simulink model "Inverters_Data"  (R2023b)
settings: Solver=FixedStepAuto  StartTime=0.0  StopTime=10.0  RelTol=1e-3
libraries: simulink x3
settings Model: Creator=cspt  LastModifiedBy=joser
settings SolverCC: AlgebraicLoopSolver=TrustRegion
settings DataIOCC: SaveOutput=off  ReturnWorkspaceOutputs=off
settings OptimizationCC: DefaultParameterBehavior=Inlined
settings DebuggingCC: UnconnectedInputMsg=warning  UnconnectedOutputMsg=warning  UnconnectedLineMsg=warning  ArithmeticOperatorsInVariantConditions=warning
settings ModelReferenceCC: EnableRefExpFcnMdlSchedulingChecks=on
settings SFSimCC: SimUseLocalCustomCode=off  CustomCodeUndefinedFunction=UseInterfaceOnly
settings RTWCC: Description=INTECRIO Real-Time Target  SystemTargetFile=irt.tlc  TemplateMakefile=irt_default_tmf  RTWUseLocalCustomCode=off
settings STFCustomTargetCC: UtilityFuncGeneration=Shared location  MatFileLogging=on  GRTInterface=on  SystemTargetFile=irt.tlc
settings GRTTargetCC: UtilityFuncGeneration=Shared location  ParMdlRefBuildCompliant=off  CompOptLevelCompliant=off  ConcurrentExecutionCompliant=off  CombineOutputUpdateFcns=off  CPPClassGenCompliant=off  GRTInterface=on  UseToolchainInfoCompliant=off  GenerateASAP2=on

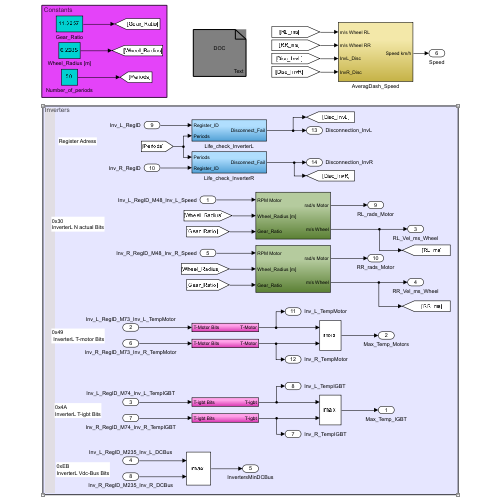
[thumbnail: Simulink's stored preview of the top-level diagram]
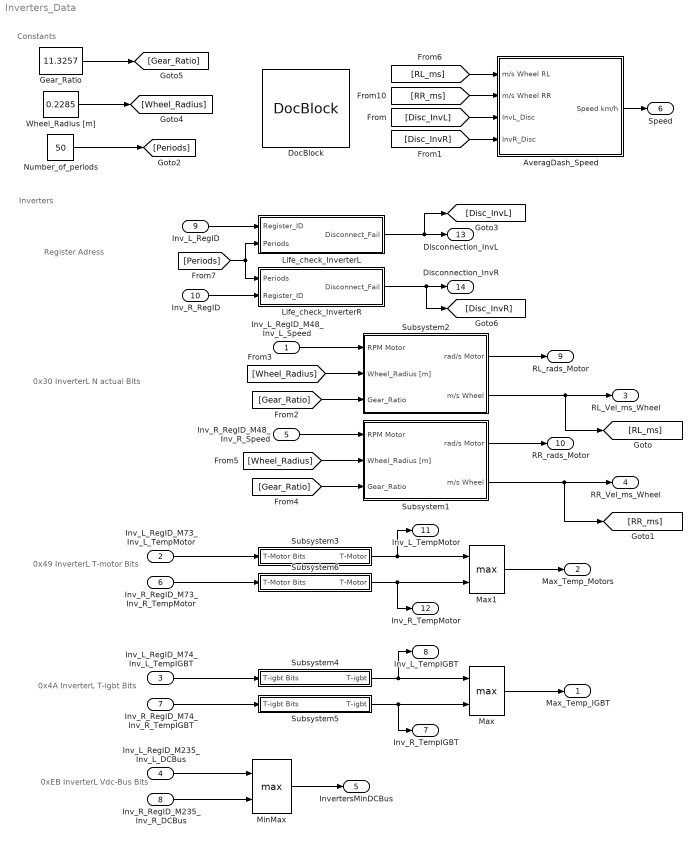
== system Inverters_Data ==
  note: Constants
  note: 0x49
      |  InverterL T-motor Bits
  note: 0x4A
      | InverterL T-igbt Bits
  note: 0xEB
      | InverterL Vdc-Bus Bits
  note: 0x30
      | InverterL N actual Bits
  note: Inverters
  note: Register Adress
  Inv_L_RegID_M48_Inv_L_Speed : Inport
  Inv_L_RegID_M73_Inv_L_TempMotor : Inport  Port=2
  Inv_L_RegID_M74_Inv_L_TempIGBT : Inport  Port=3
  Inv_L_RegID_M235_Inv_L_DCBus : Inport  Port=4
  Inv_R_RegID_M48_Inv_R_Speed : Inport  Port=5
  Inv_R_RegID_M73_Inv_R_TempMotor : Inport  Port=6
  Inv_R_RegID_M74_Inv_R_TempIGBT : Inport  Port=7
  Inv_R_RegID_M235_Inv_R_DCBus : Inport  Port=8
  Inv_L_RegID : Inport  Port=9
  Inv_R_RegID : Inport  Port=10
  AveragDash_Speed : Subsystem
  DocBlock : simulink/Model-Wide Utilities/DocBlock  DocumentType=Text
      content=|
      | Our Bamocar Inverters communicate with the environment in bits.
      | A maximum number of bits (32767) is selected to correspond to a maximum
      | number of current, RPM, etc., which would be equivalent to 100%, but it
      | can send or receive a greater number of bits.
      |
      | The 3 currents (Iq, Iactual, Icmd) conversion are done on the Database:
      | 400 / 1070 = 0.3738317757...
      |
      | The "Inv_X_DCBus" conversion is done on the Database: 0.03125
      | The function of Bits - VoltageDCBus is linear, so we need the slope:
      | f(Bits) = Voltage    f(22000 Bits) = 700 V     f(14000 Bits) = 450 V
      | (700 - 450) / (22000 - 14000) = 0.03125
      |
      | The "Inv_X_Speed" conversion is done on the Database:
      | 'N-100%' (RPMmax) / 32767 (Bits_max) = 0.18311057
      | RPMmax is the speed limit selected on the N-Drive Software (talk with Powertrain)
      |
      | The Motor Temp is done in the Database: TempM * 0.03282 - 114.92892
      |
      | The IGBT & Motor Temps are complex, so the conversions are done on the
      | Simulink. The Powertrain Department provided us with a Bits - Temp lookup
      | table. The Bits are on CAN1 (send by the Inverters) and the ºC are send
      | through CAN2.
      |
      | All values with understandable units are at CAN1, Message:
      | AP_Inverter_X_Tx (0xB5 & 0xB6),
      | but the IGBT & Motor Temps (ºC) are at CAN2:
      | MEAS_ETAS_Inverter_X_Data (0xD2 & 0xD3).
  Gear_Ratio : Constant  Value=11.3257
  Life_check_InverterL : Subsystem
  Life_check_InverterR : Subsystem
  Max : MinMax  Function=max  Inputs=2
  Max1 : MinMax  Function=max  Inputs=2
  MinMax : MinMax  Function=max  Inputs=2
  Number_of_periods : Constant  Value=50
  Subsystem1 : Subsystem
  Subsystem2 : Subsystem
  Subsystem3 : Subsystem
  Subsystem4 : Subsystem
  Subsystem5 : Subsystem
  Subsystem6 : Subsystem
  Wheel_Radius [m] : Constant  Value=0.2285
  Max_Temp_IGBT : Outport  VectorParamsAs1DForOutWhenUnconnected=off
  Max_Temp_Motors : Outport  Port=2  VectorParamsAs1DForOutWhenUnconnected=off
  RL_Vel_ms_Wheel : Outport  Port=3  VectorParamsAs1DForOutWhenUnconnected=off
  RR_Vel_ms_Wheel : Outport  Port=4  VectorParamsAs1DForOutWhenUnconnected=off
  InvertersMinDCBus : Outport  Port=5  VectorParamsAs1DForOutWhenUnconnected=off
  Speed : Outport  Port=6  VectorParamsAs1DForOutWhenUnconnected=off
  Inv_R_TempIGBT : Outport  Port=7  VectorParamsAs1DForOutWhenUnconnected=off
  Inv_L_TempIGBT : Outport  Port=8  VectorParamsAs1DForOutWhenUnconnected=off
  RL_rads_Motor : Outport  Port=9  VectorParamsAs1DForOutWhenUnconnected=off
  RR_rads_Motor : Outport  Port=10  VectorParamsAs1DForOutWhenUnconnected=off
  Inv_L_TempMotor : Outport  Port=11
  Inv_R_TempMotor : Outport  Port=12
  Disconnection_InvL : Outport  Port=13  VectorParamsAs1DForOutWhenUnconnected=off
  Disconnection_InvR : Outport  Port=14  VectorParamsAs1DForOutWhenUnconnected=off
  wires:
  Max1/1 -> Max_Temp_Motors/1
  [RR_ms] -> AveragDash_Speed/2(m/s Wheel RR)
  Subsystem2/2(m/s Wheel) -> [RL_ms], RL_Vel_ms_Wheel/1
  Subsystem4/1(T-igbt) -> Inv_L_TempIGBT/1, Max/1
  Subsystem1/2(m/s Wheel) -> RR_Vel_ms_Wheel/1, [RR_ms]
  Inv_L_RegID_M74_Inv_L_TempIGBT/1 -> Subsystem4/1(T-igbt Bits)
  [RL_ms] -> AveragDash_Speed/1(m/s Wheel RL)
  AveragDash_Speed/1(Speed km/h) -> Speed/1
  MinMax/1 -> InvertersMinDCBus/1
  Inv_R_RegID_M74_Inv_R_TempIGBT/1 -> Subsystem5/1(T-igbt Bits)
  Max/1 -> Max_Temp_IGBT/1
  Subsystem5/1(T-igbt) -> Inv_R_TempIGBT/1, Max/2
  Inv_L_RegID_M235_Inv_L_DCBus/1 -> MinMax/1
  Inv_R_RegID_M235_Inv_R_DCBus/1 -> MinMax/2
  Subsystem1/1(rad/s Motor) -> RR_rads_Motor/1
  Subsystem2/1(rad/s Motor) -> RL_rads_Motor/1
  Wheel_Radius [m]/1 -> [Wheel_Radius]
  Gear_Ratio/1 -> [Gear_Ratio]
  Inv_R_RegID_M48_Inv_R_Speed/1 -> Subsystem1/1(RPM Motor)
  [Gear_Ratio] -> Subsystem2/3(Gear_Ratio)
  [Wheel_Radius] -> Subsystem2/2(Wheel_Radius [m])
  Inv_L_RegID_M48_Inv_L_Speed/1 -> Subsystem2/1(RPM Motor)
  [Gear_Ratio] -> Subsystem1/3(Gear_Ratio)
  [Wheel_Radius] -> Subsystem1/2(Wheel_Radius [m])
  Life_check_InverterR/1(Disconnect_Fail) -> Disconnection_InvR/1, [Disc_InvR]
  Life_check_InverterL/1(Disconnect_Fail) -> Disconnection_InvL/1, [Disc_InvL]
  Inv_L_RegID/1 -> Life_check_InverterL/1(Register_ID)
  Inv_R_RegID/1 -> Life_check_InverterR/2(Register_ID)
  [Periods] -> Life_check_InverterR/1(Periods), Life_check_InverterL/2(Periods)
  Number_of_periods/1 -> [Periods]
  Inv_L_RegID_M73_Inv_L_TempMotor/1 -> Subsystem3/1(T-Motor Bits)
  Subsystem3/1(T-Motor) -> Max1/1, Inv_L_TempMotor/1
  Subsystem6/1(T-Motor) -> Inv_R_TempMotor/1, Max1/2
  Inv_R_RegID_M73_Inv_R_TempMotor/1 -> Subsystem6/1(T-Motor Bits)
  [Disc_InvR] -> AveragDash_Speed/4(InvR_Disc)
  [Disc_InvL] -> AveragDash_Speed/3(InvL_Disc)

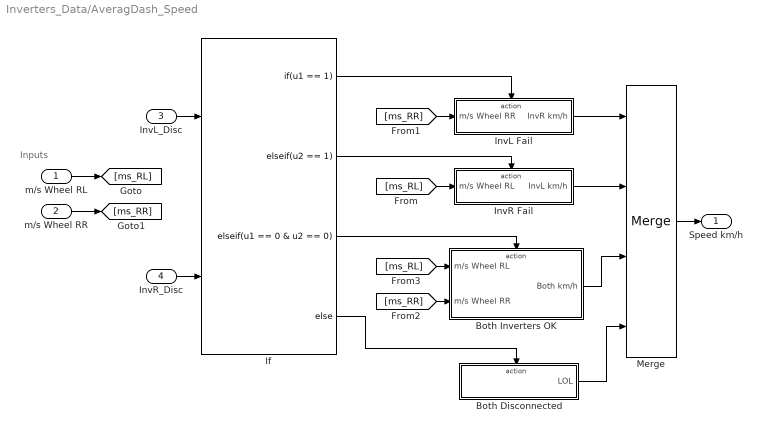
== system Inverters_Data/AveragDash_Speed ==
  note: Inputs
  m/s Wheel RL : Inport
  m/s Wheel RR : Inport  Port=2
  InvL_Disc : Inport  Port=3
  InvR_Disc : Inport  Port=4
  Both Disconnected : Subsystem  TreatAsAtomicUnit=on
  Both Inverters OK : Subsystem  TreatAsAtomicUnit=on
  If : If  NumInputs=2  IfExpression=u1 == 1  ElseIfExpressions=u2 == 1, u1 == 0 & u2 == 0
  InvL Fail : Subsystem  TreatAsAtomicUnit=on
  InvR Fail : Subsystem  TreatAsAtomicUnit=on
  Merge : Merge  Inputs=4
  Speed km/h : Outport  VectorParamsAs1DForOutWhenUnconnected=off
  wires:
  m/s Wheel RL/1 -> [ms_RL]
  m/s Wheel RR/1 -> [ms_RR]
  InvL_Disc/1 -> If/1
  InvR_Disc/1 -> If/2
  Merge/1 -> Speed km/h/1
  If/1 -> InvL Fail/Action
  If/2 -> InvR Fail/Action
  InvL Fail/1(InvR km/h) -> Merge/1
  InvR Fail/1(InvL km/h) -> Merge/2
  If/3 -> Both Inverters OK/Action
  Both Inverters OK/1(Both km/h) -> Merge/3
  [ms_RL] -> InvR Fail/1(m/s Wheel RL)
  [ms_RR] -> InvL Fail/1(m/s Wheel RR)
  [ms_RR] -> Both Inverters OK/2(m/s Wheel RR)
  [ms_RL] -> Both Inverters OK/1(m/s Wheel RL)
  If/4 -> Both Disconnected/Action
  Both Disconnected/1(LOL) -> Merge/4

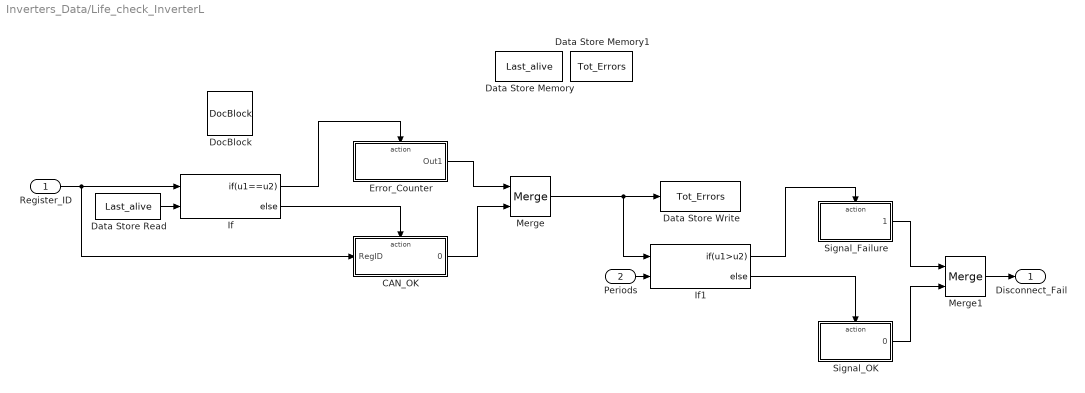
== system Inverters_Data/Life_check_InverterL ==
  Register_ID : Inport
  Periods : Inport  Port=2
  CAN_OK : Subsystem  TreatAsAtomicUnit=on
  Data Store Memory : DataStoreMemory  DataStoreName=Last_alive  ReadBeforeWriteMsg=warning  WriteAfterWriteMsg=warning  WriteAfterReadMsg=warning  ShowAdditionalParam=off
  Data Store Memory1 : DataStoreMemory  DataStoreName=Tot_Errors  ReadBeforeWriteMsg=warning  WriteAfterWriteMsg=warning  WriteAfterReadMsg=warning  ShowAdditionalParam=off
  Data Store Read : DataStoreRead  DataStoreName=Last_alive  IndexOptions=Index vector (dialog)  Indices=1  OutputSizes=1
  Data Store Write : DataStoreWrite  DataStoreName=Tot_Errors  IndexOptions=Index vector (dialog)  Indices=1  OutputSizes=1
  DocBlock : simulink/Model-Wide Utilities/DocBlock  DocumentType=Text
      content=|
      | The 'Inverters_Data' Simulink module is computed every 3ms by the ETAS.
      |
      | An Inverter is considered disconnected if the same value is obtained
      | from it for more than X seconds:
      | 0,003sec (Simulink computed) * P periods ('Periods' constant) = X seconds
      |
      | The Register Adress (RegID) has to modify its value every 3ms, because it
      | sends diferents signals every 3ms (multiplexed).
      |
      | This type of disconnection checks if there has been an error for more than
      | X seconds: STARTS counting since that first 'error' output. The important
      | thing about the Inverters' disconnections is the time it has been
      | disconnected, that's why we do it after checking the error.
      |
      | I've done some tests, and when I disconnect and then reconnect the
      | inverter, the RegID changes to a different period than before (3ms). I
      | don't understand why this happens.
      |
      | If we compute this subsystem at 'Disconnections', the ETAS would check the
      | alive every 25ms (when the RegID could be same as before), instead of every
      | 3ms (the RegID changes every 3ms).
      |
      | There's a an error -> Start counting errors -> Errors persist through X
      | periods -> Sensor disconnection
  Error_Counter : Subsystem  TreatAsAtomicUnit=on
  If : If  NumInputs=2  IfExpression=u1==u2
  If1 : If  NumInputs=2  IfExpression=u1>u2
  Merge : Merge
  Merge1 : Merge
  Signal_Failure : Subsystem  TreatAsAtomicUnit=on
  Signal_OK : Subsystem  TreatAsAtomicUnit=on
  Disconnect_Fail : Outport  VectorParamsAs1DForOutWhenUnconnected=off
  wires:
  Data Store Read/1 -> If/2
  If/2 -> CAN_OK/Action
  CAN_OK/1(0) -> Merge/2
  Register_ID/1 -> If/1, CAN_OK/1(RegID)
  If/1 -> Error_Counter/Action
  Error_Counter/1(Out1) -> Merge/1
  Merge/1 -> Data Store Write/1, If1/1
  If1/2 -> Signal_OK/Action
  Periods/1 -> If1/2
  Signal_Failure/1(1) -> Merge1/1
  If1/1 -> Signal_Failure/Action
  Signal_OK/1(0) -> Merge1/2
  Merge1/1 -> Disconnect_Fail/1

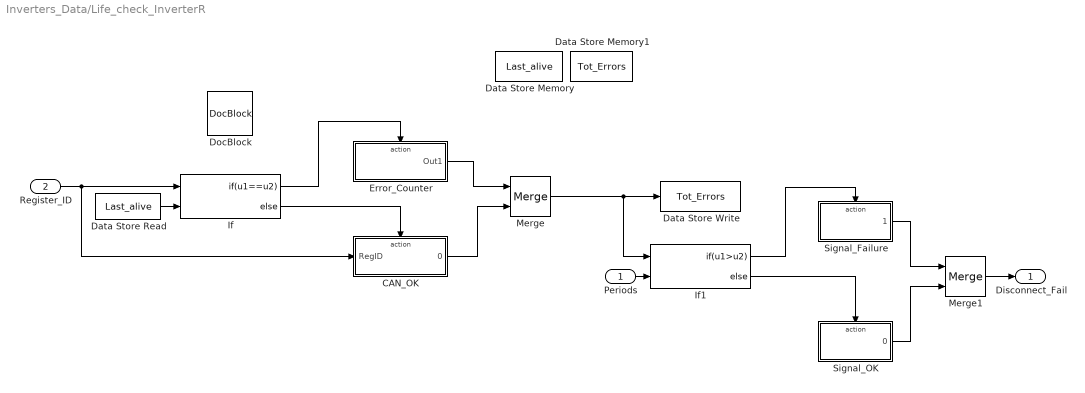
== system Inverters_Data/Life_check_InverterR ==
  Periods : Inport
  Register_ID : Inport  Port=2
  CAN_OK : Subsystem  TreatAsAtomicUnit=on
  Data Store Memory : DataStoreMemory  DataStoreName=Last_alive  ReadBeforeWriteMsg=warning  WriteAfterWriteMsg=warning  WriteAfterReadMsg=warning  ShowAdditionalParam=off
  Data Store Memory1 : DataStoreMemory  DataStoreName=Tot_Errors  ReadBeforeWriteMsg=warning  WriteAfterWriteMsg=warning  WriteAfterReadMsg=warning  ShowAdditionalParam=off
  Data Store Read : DataStoreRead  DataStoreName=Last_alive  IndexOptions=Index vector (dialog)  Indices=1  OutputSizes=1
  Data Store Write : DataStoreWrite  DataStoreName=Tot_Errors  IndexOptions=Index vector (dialog)  Indices=1  OutputSizes=1
  DocBlock : simulink/Model-Wide Utilities/DocBlock  DocumentType=Text
      content=|
      | The 'Inverters_Data' Simulink module is computed every 3ms by the ETAS.
      |
      | An Inverter is considered disconnected if the same value is obtained
      | from it for more than X seconds:
      | 0,003sec (Simulink computed) * P periods ('Periods' constant) = X seconds
      |
      | The Register Adress (RegID) has to modify its value every 3ms, because it
      | sends diferents signals every 3ms (multiplexed).
      |
      | This type of disconnection checks if there has been an error for more than
      | X seconds: STARTS counting since that first 'error' output. The important
      | thing about the Inverters' disconnections is the time it has been
      | disconnected, that's why we do it after checking the error.
      |
      | I've done some tests, and when I disconnect and then reconnect the
      | inverter, the RegID changes to a different period than before (3ms). I
      | don't understand why this happens.
      |
      | If we compute this subsystem at 'Disconnections', the ETAS would check the
      | alive every 25ms (when the RegID could be same as before), instead of every
      | 3ms (the RegID changes every 3ms).
      |
      | There's a an error -> Start counting errors -> Errors persist through X
      | periods -> Sensor disconnection
  Error_Counter : Subsystem  TreatAsAtomicUnit=on
  If : If  NumInputs=2  IfExpression=u1==u2
  If1 : If  NumInputs=2  IfExpression=u1>u2
  Merge : Merge
  Merge1 : Merge
  Signal_Failure : Subsystem  TreatAsAtomicUnit=on
  Signal_OK : Subsystem  TreatAsAtomicUnit=on
  Disconnect_Fail : Outport  VectorParamsAs1DForOutWhenUnconnected=off
  wires:
  Data Store Read/1 -> If/2
  If/2 -> CAN_OK/Action
  CAN_OK/1(0) -> Merge/2
  Register_ID/1 -> If/1, CAN_OK/1(RegID)
  If/1 -> Error_Counter/Action
  Error_Counter/1(Out1) -> Merge/1
  Merge/1 -> Data Store Write/1, If1/1
  If1/2 -> Signal_OK/Action
  Periods/1 -> If1/2
  Signal_Failure/1(1) -> Merge1/1
  If1/1 -> Signal_Failure/Action
  Signal_OK/1(0) -> Merge1/2
  Merge1/1 -> Disconnect_Fail/1

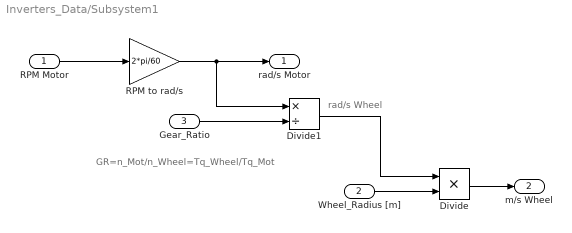
== system Inverters_Data/Subsystem1 ==
  note: rad/s Wheel
  note: GR=n_Mot/n_Wheel=Tq_Wheel/Tq_Mot
  RPM Motor : Inport
  Wheel_Radius [m] : Inport  Port=2
  Gear_Ratio : Inport  Port=3
  Divide : Product  Inputs=**
  Divide1 : Product  Inputs=*/
  RPM to rad/s : Gain  Gain=2*pi/60
  rad/s Motor : Outport  VectorParamsAs1DForOutWhenUnconnected=off
  m/s Wheel : Outport  Port=2
  wires:
  RPM to rad/s/1 -> Divide1/1, rad/s Motor/1
  Divide1/1 -> Divide/1
  Wheel_Radius [m]/1 -> Divide/2
  Divide/1 -> m/s Wheel/1
  Gear_Ratio/1 -> Divide1/2
  RPM Motor/1 -> RPM to rad/s/1

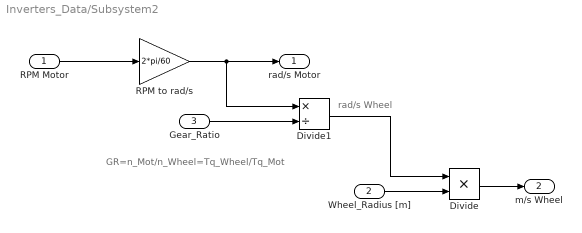
== system Inverters_Data/Subsystem2 ==
  note: rad/s Wheel
  note: GR=n_Mot/n_Wheel=Tq_Wheel/Tq_Mot
  RPM Motor : Inport
  Wheel_Radius [m] : Inport  Port=2
  Gear_Ratio : Inport  Port=3
  Divide : Product  Inputs=**
  Divide1 : Product  Inputs=*/
  RPM to rad/s : Gain  Gain=2*pi/60
  rad/s Motor : Outport  VectorParamsAs1DForOutWhenUnconnected=off
  m/s Wheel : Outport  Port=2
  wires:
  RPM to rad/s/1 -> Divide1/1, rad/s Motor/1
  Divide1/1 -> Divide/1
  Wheel_Radius [m]/1 -> Divide/2
  Divide/1 -> m/s Wheel/1
  Gear_Ratio/1 -> Divide1/2
  RPM Motor/1 -> RPM to rad/s/1

== system Inverters_Data/Subsystem3 ==
  T-Motor Bits : Inport
  1-D Lookup Table : Lookup_n-D  NumberOfTableDimensions=1  BreakpointsForDimension1=[3788.961224,3945.578464,4023.494666,4178.542234,4249.749706,4403.26785,4555.739546,4631.582976,4701.360096,4851.779144,5001.151744,5143.792394,5291.112346,5437.38585,5504.543754,5649.287834,5721.267456,5792.985466,5930.169416,6001.122714,6071.8144,6142.244474,6207.02465,6276.951624,6346.616986,6416.020736,6548.754186,6617.393224,6712,6816.5304,6868.5634,7075.1474,7126.4064,7228.46,7279.2546,7480.885,7530.9056,7580.7714,7680.0386,7729.44,7778.6866,7827.7784,7925.4976,7974.125,8022.5976,8119.0784,8262.6386,8357.5714,8404.8056,8592.1944,8638.6546,8822.9474,8914.165,9004.7634]  Table=[1.31,7.1,9.99,15.2,18.1,23.9,29.1,32,34.9,40.1,45.9,50.5,55.7,60.4,62.7,66.7,69,71.4,75.4,77.7,80,81.8,83.5,85.2,87,88.7,93.3,95.1,100,101,103,108,110,112,114,119,121,123,125,126,128,130,132,133,135,137,143,144,146,152,154,159,165,168]  InternalRulePriority=Speed  RndMeth=Simplest
  T-Motor : Outport  VectorParamsAs1DForOutWhenUnconnected=off
  wires:
  T-Motor Bits/1 -> 1-D Lookup Table/1
  1-D Lookup Table/1 -> T-Motor/1

== system Inverters_Data/Subsystem4 ==
  T-igbt Bits : Inport
  1-D Lookup Table : Lookup_n-D  NumberOfTableDimensions=1  BreakpointsForDimension1="[15610\t15640\t15680\t15730\t15780\t15830\t15880\t15910\t15960\t16000\t16070\t16130\t16180\t16250\t16320\t16390\t16440\t16520\t16590\t16670\t16740\t16810\t16890\t16980\t17060\t17150\t17230\t17330\t17440\t17520\t17620\t17720\t17830\t17930\t18030\t18130\t18250\t18350\t18470\t18590\t18690\t18810\t18940\t19060\t19180\t19300\t19420\t19550\t19690\t19810\t19940\t20080\t20210\t20330\t20470\t20600\t20740\t20870\t21020\t21160\t21300\t21410\t21550\t21680\t21820\t21960\t22110\t22240\t22380\t22510\t22650\t22790\t22920\t23060\t23190\t23330\t23460\t23580\t23720\t23830\t23970\t24090\t24210\t24340\t24460\t24580\t24700\t24820\t24930\t25050\t25170\t25290\t25390\t25510\t25630\t25730\t25830\t25930\t26040\t26140]"  Table="[-10.01\t-8.877\t-7.746\t-6.701\t-5.57\t-4.439\t-3.307\t-2.263\t-1.131\t0\t1.131\t2.176\t3.307\t4.439\t5.57\t6.701\t7.746\t8.877\t10.01\t11.14\t12.18\t13.32\t14.45\t15.58\t16.62\t17.75\t18.89\t20.02\t21.06\t22.19\t23.32\t24.46\t25.59\t26.63\t27.76\t28.89\t30.03\t31.07\t32.20\t33.33\t34.46\t35.51\t36.64\t37.77\t38.90\t40.03\t41.08\t42.21\t43.34\t44.47\t45.52\t46.65\t47.78\t48.91\t49.96\t51.09\t52.22\t53.35\t54.48\t55.53\t56.66\t57.79\t58.92\t59.97\t61.10\t62.23\t63.36\t64.40\t65.54\t66.67\t67.80\t68.93\t69.97\t71.11\t72.24\t73.37\t74.41\t75.54\t76.68\t77.81\t78.85\t79.98\t81.11\t82.25\t83.29\t84.42\t85.55\t86.68\t87.82\t88.86\t89.99\t91.12\t92.25\t93.30\t94.43\t95.56\t96.69\t97.74\t98.87\t100]"  InternalRulePriority=Speed  RndMeth=Simplest
  T-igbt : Outport  VectorParamsAs1DForOutWhenUnconnected=off
  wires:
  T-igbt Bits/1 -> 1-D Lookup Table/1
  1-D Lookup Table/1 -> T-igbt/1

== system Inverters_Data/Subsystem5 ==
  T-igbt Bits : Inport
  1-D Lookup Table : Lookup_n-D  NumberOfTableDimensions=1  BreakpointsForDimension1="[15610\t15640\t15680\t15730\t15780\t15830\t15880\t15910\t15960\t16000\t16070\t16130\t16180\t16250\t16320\t16390\t16440\t16520\t16590\t16670\t16740\t16810\t16890\t16980\t17060\t17150\t17230\t17330\t17440\t17520\t17620\t17720\t17830\t17930\t18030\t18130\t18250\t18350\t18470\t18590\t18690\t18810\t18940\t19060\t19180\t19300\t19420\t19550\t19690\t19810\t19940\t20080\t20210\t20330\t20470\t20600\t20740\t20870\t21020\t21160\t21300\t21410\t21550\t21680\t21820\t21960\t22110\t22240\t22380\t22510\t22650\t22790\t22920\t23060\t23190\t23330\t23460\t23580\t23720\t23830\t23970\t24090\t24210\t24340\t24460\t24580\t24700\t24820\t24930\t25050\t25170\t25290\t25390\t25510\t25630\t25730\t25830\t25930\t26040\t26140]"  Table="[-10.01\t-8.877\t-7.746\t-6.701\t-5.57\t-4.439\t-3.307\t-2.263\t-1.131\t0\t1.131\t2.176\t3.307\t4.439\t5.57\t6.701\t7.746\t8.877\t10.01\t11.14\t12.18\t13.32\t14.45\t15.58\t16.62\t17.75\t18.89\t20.02\t21.06\t22.19\t23.32\t24.46\t25.59\t26.63\t27.76\t28.89\t30.03\t31.07\t32.20\t33.33\t34.46\t35.51\t36.64\t37.77\t38.90\t40.03\t41.08\t42.21\t43.34\t44.47\t45.52\t46.65\t47.78\t48.91\t49.96\t51.09\t52.22\t53.35\t54.48\t55.53\t56.66\t57.79\t58.92\t59.97\t61.10\t62.23\t63.36\t64.40\t65.54\t66.67\t67.80\t68.93\t69.97\t71.11\t72.24\t73.37\t74.41\t75.54\t76.68\t77.81\t78.85\t79.98\t81.11\t82.25\t83.29\t84.42\t85.55\t86.68\t87.82\t88.86\t89.99\t91.12\t92.25\t93.30\t94.43\t95.56\t96.69\t97.74\t98.87\t100]"  InternalRulePriority=Speed  RndMeth=Simplest
  T-igbt : Outport  VectorParamsAs1DForOutWhenUnconnected=off
  wires:
  T-igbt Bits/1 -> 1-D Lookup Table/1
  1-D Lookup Table/1 -> T-igbt/1

== system Inverters_Data/Subsystem6 ==
  T-Motor Bits : Inport
  1-D Lookup Table : Lookup_n-D  NumberOfTableDimensions=1  BreakpointsForDimension1=[3788.961224,3945.578464,4023.494666,4178.542234,4249.749706,4403.26785,4555.739546,4631.582976,4701.360096,4851.779144,5001.151744,5143.792394,5291.112346,5437.38585,5504.543754,5649.287834,5721.267456,5792.985466,5930.169416,6001.122714,6071.8144,6142.244474,6207.02465,6276.951624,6346.616986,6416.020736,6548.754186,6617.393224,6712,6816.5304,6868.5634,7075.1474,7126.4064,7228.46,7279.2546,7480.885,7530.9056,7580.7714,7680.0386,7729.44,7778.6866,7827.7784,7925.4976,7974.125,8022.5976,8119.0784,8262.6386,8357.5714,8404.8056,8592.1944,8638.6546,8822.9474,8914.165,9004.7634]  Table=[1.31,7.1,9.99,15.2,18.1,23.9,29.1,32,34.9,40.1,45.9,50.5,55.7,60.4,62.7,66.7,69,71.4,75.4,77.7,80,81.8,83.5,85.2,87,88.7,93.3,95.1,100,101,103,108,110,112,114,119,121,123,125,126,128,130,132,133,135,137,143,144,146,152,154,159,165,168]  InternalRulePriority=Speed  RndMeth=Simplest
  T-Motor : Outport  VectorParamsAs1DForOutWhenUnconnected=off
  wires:
  T-Motor Bits/1 -> 1-D Lookup Table/1
  1-D Lookup Table/1 -> T-Motor/1

== system Inverters_Data/AveragDash_Speed/Both Disconnected ==
  Action Port : ActionPort  ActionPortLabel=else
  Constant : Constant  Value=69
  LOL : Outport  VectorParamsAs1DForOutWhenUnconnected=off
  wires:
  Constant/1 -> LOL/1

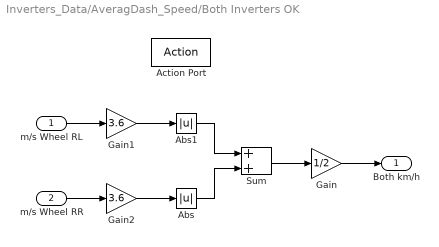
== system Inverters_Data/AveragDash_Speed/Both Inverters OK ==
  m/s Wheel RL : Inport
  m/s Wheel RR : Inport  Port=2
  Action Port : ActionPort  ActionPortLabel=elseif( u1 == 0 & u2 == 0)
  Abs : Abs  SaturateOnIntegerOverflow=off
  Abs1 : Abs  SaturateOnIntegerOverflow=off
  Gain : Gain  Gain=1/2
  Gain1 : Gain  Gain=3.6
  Gain2 : Gain  Gain=3.6
  Sum : Sum
  Both km/h : Outport  VectorParamsAs1DForOutWhenUnconnected=off
  wires:
  Abs1/1 -> Sum/1
  Abs/1 -> Sum/2
  m/s Wheel RR/1 -> Gain2/1
  Gain2/1 -> Abs/1
  Gain1/1 -> Abs1/1
  m/s Wheel RL/1 -> Gain1/1
  Sum/1 -> Gain/1
  Gain/1 -> Both km/h/1

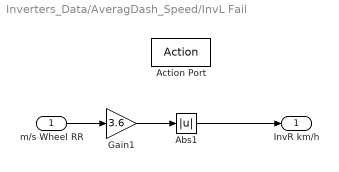
== system Inverters_Data/AveragDash_Speed/InvL Fail ==
  m/s Wheel RR : Inport
  Action Port : ActionPort  ActionPortLabel=if(u1 == 1)
  Abs1 : Abs  SaturateOnIntegerOverflow=off
  Gain1 : Gain  Gain=3.6
  InvR km/h : Outport  VectorParamsAs1DForOutWhenUnconnected=off
  wires:
  Gain1/1 -> Abs1/1
  m/s Wheel RR/1 -> Gain1/1
  Abs1/1 -> InvR km/h/1

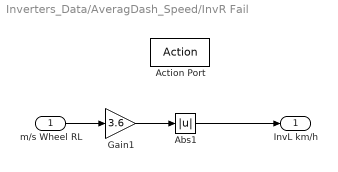
== system Inverters_Data/AveragDash_Speed/InvR Fail ==
  m/s Wheel RL : Inport
  Action Port : ActionPort  ActionPortLabel=elseif(u2 == 1)
  Abs1 : Abs  SaturateOnIntegerOverflow=off
  Gain1 : Gain  Gain=3.6
  InvL km/h : Outport  VectorParamsAs1DForOutWhenUnconnected=off
  wires:
  Gain1/1 -> Abs1/1
  m/s Wheel RL/1 -> Gain1/1
  Abs1/1 -> InvL km/h/1

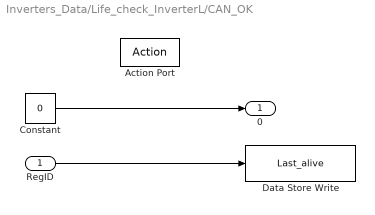
== system Inverters_Data/Life_check_InverterL/CAN_OK ==
  RegID : Inport
  Action Port : ActionPort  ActionPortLabel=else
  Constant : Constant  Value=0
  Data Store Write : DataStoreWrite  DataStoreName=Last_alive  IndexOptions=Index vector (dialog)  Indices=1  OutputSizes=1
  0 : Outport  VectorParamsAs1DForOutWhenUnconnected=off
  wires:
  Constant/1 -> 0/1
  RegID/1 -> Data Store Write/1

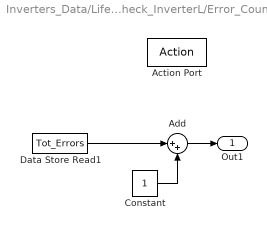
== system Inverters_Data/Life_check_InverterL/Error_Counter ==
  Action Port : ActionPort  ActionPortLabel=if(u1==u2)
  Add : Sum  Inputs=|++
  Constant : Constant
  Data Store Read1 : DataStoreRead  DataStoreName=Tot_Errors  IndexOptions=Index vector (dialog)  Indices=1  OutputSizes=1
  Out1 : Outport  VectorParamsAs1DForOutWhenUnconnected=off
  wires:
  Constant/1 -> Add/2
  Data Store Read1/1 -> Add/1
  Add/1 -> Out1/1

== system Inverters_Data/Life_check_InverterL/Signal_Failure ==
  Action Port : ActionPort  ActionPortLabel=if(u1>u2)
  Constant : Constant
  1 : Outport  VectorParamsAs1DForOutWhenUnconnected=off
  wires:
  Constant/1 -> 1/1

== system Inverters_Data/Life_check_InverterL/Signal_OK ==
  Action Port : ActionPort  ActionPortLabel=else
  Constant : Constant  Value=0
  0 : Outport  VectorParamsAs1DForOutWhenUnconnected=off
  wires:
  Constant/1 -> 0/1

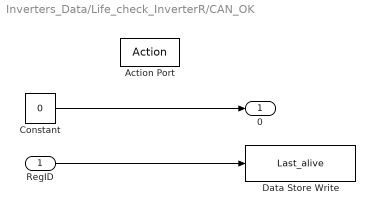
== system Inverters_Data/Life_check_InverterR/CAN_OK ==
  RegID : Inport
  Action Port : ActionPort  ActionPortLabel=else
  Constant : Constant  Value=0
  Data Store Write : DataStoreWrite  DataStoreName=Last_alive  IndexOptions=Index vector (dialog)  Indices=1  OutputSizes=1
  0 : Outport  VectorParamsAs1DForOutWhenUnconnected=off
  wires:
  Constant/1 -> 0/1
  RegID/1 -> Data Store Write/1

== system Inverters_Data/Life_check_InverterR/Error_Counter ==
  Action Port : ActionPort  ActionPortLabel=if(u1==u2)
  Add : Sum  Inputs=|++
  Constant : Constant
  Data Store Read1 : DataStoreRead  DataStoreName=Tot_Errors  IndexOptions=Index vector (dialog)  Indices=1  OutputSizes=1
  Out1 : Outport  VectorParamsAs1DForOutWhenUnconnected=off
  wires:
  Constant/1 -> Add/2
  Data Store Read1/1 -> Add/1
  Add/1 -> Out1/1

== system Inverters_Data/Life_check_InverterR/Signal_Failure ==
  Action Port : ActionPort  ActionPortLabel=if(u1>u2)
  Constant : Constant
  1 : Outport  VectorParamsAs1DForOutWhenUnconnected=off
  wires:
  Constant/1 -> 1/1

== system Inverters_Data/Life_check_InverterR/Signal_OK ==
  Action Port : ActionPort  ActionPortLabel=else
  Constant : Constant  Value=0
  0 : Outport  VectorParamsAs1DForOutWhenUnconnected=off
  wires:
  Constant/1 -> 0/1
